simulink model "Demo2_P2A1"  (R2023a)
settings: Solver=VariableStepAuto  StartTime=0.0  StopTime=5  RelTol=1e-3
settings Model: Creator=rqouta  LastModifiedBy=rqouta

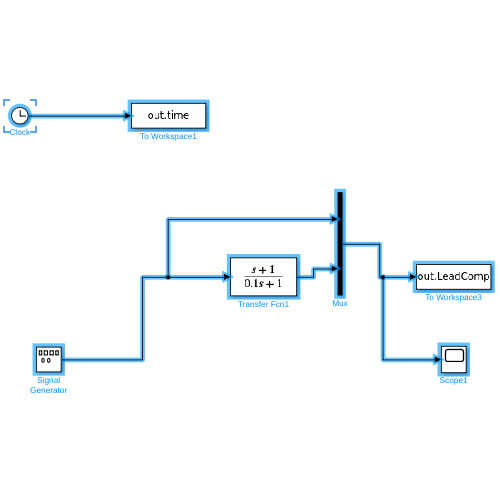
[thumbnail: Simulink's stored preview of the top-level diagram]
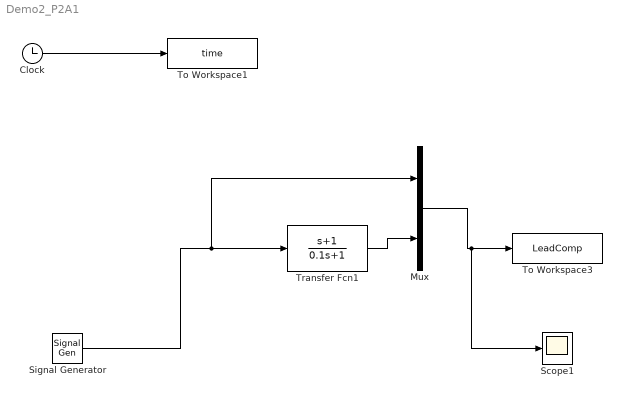
== system Demo2_P2A1 ==
  Clock : Clock
  Mux : Mux  Inputs=2
  Scope1 : Scope
  Signal Generator : SignalGenerator  WaveForm=square  Frequency=0.2
  To Workspace1 : ToWorkspace  VariableName=time  SampleTime=-1
  To Workspace3 : ToWorkspace  VariableName=LeadComp  SampleTime=-1
  Transfer Fcn1 : TransferFcn  Numerator=[1 1]  Denominator=[0.1 1]
  wires:
  Clock/1 -> To Workspace1/1
  Signal Generator/1 -> Mux/1, Transfer Fcn1/1
  Mux/1 -> Scope1/1, To Workspace3/1
  Transfer Fcn1/1 -> Mux/2
